simulink model "Stator_Resistance_tunning_induction_motor_NIKHIL_TYAGI"  (R2023b)
settings: Solver=ode4  StartTime=0.0  StopTime=5  RelTol=1e-3
libraries: spsabctoAlphaBetaZeroLib x3, spsStairGeneratorLib x3, slpidlib x3, spsThreePhaseVIMeasurementLib x2, spsAsynchronousMachineSIUnitsLib x1, spsSeriesRLCBranchLib x1, spsUniversalBridgeLib x1, spsThreePhaseSourceLib x1, spsSVPWMGenerator2LevelLib x1, spsTwoLevelConverterLib x1, spsVoltageMeasurementLib x1, spsdq0toabcLib x1
settings Model: Creator=tyagi  LastModifiedBy=tyagi_av27qbo
settings OptimizationCC: ReuseModelBlockBuffer=off

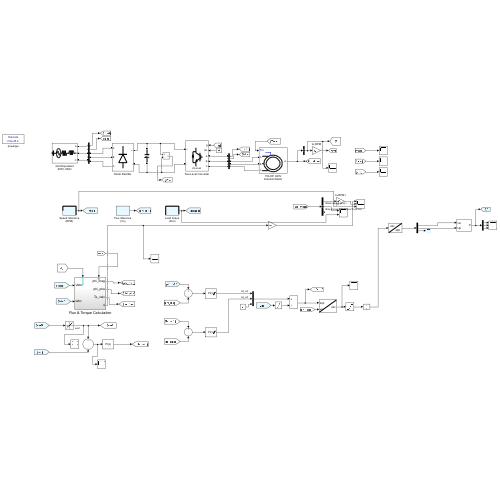
[thumbnail: Simulink's stored preview of the top-level diagram]
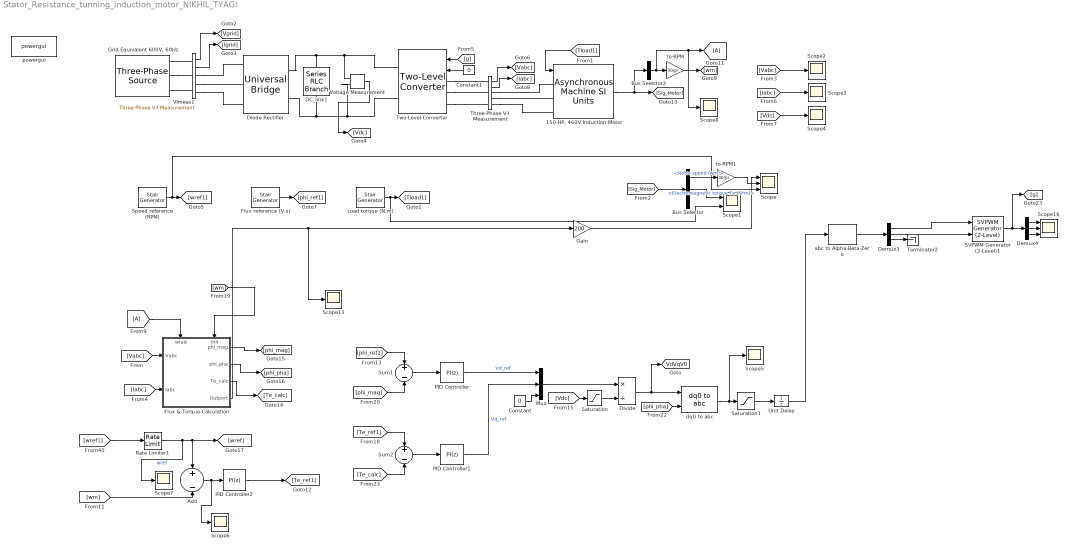
== system Stator_Resistance_tunning_induction_motor_NIKHIL_TYAGI ==
  "150-HP, 460V Induction Motor" : spsAsynchronousMachineSIUnitsLib/Asynchronous Machine SI Units  RotorType=Squirrel-cage  PresetModel=No  MechanicalLoad=Torque Tm  ShowDetailedParameters=on  ReferenceFrame=Stationary  Units=SI  MeasurementBus=off  NominalParameters="[ 111900  460  60]"  VoltageRatio=1  Stator=[0.0302,0.000283]  Rotor=[0.0302,0.000283]  Cage1=[ 0.022 0.226/377]  Cage2=[ 0.022 0.226/377]  Lm=0.01095  Mechanical=[2,0.02154,2]  PolePairs=2  InitialConditions=[1,0,0,0,0,0,0,0]  SimulateSaturation=off  Saturation=[0 0;0 0]  LoadFlowParameters=0  TsPowergui=0  TsBlock=-1  IterativeModel=Trapezoidal non iterative  IterativeDiscreteModel=Trapezoidal robust  Pmec=0  mask(Asynchronous Machine){}
      settings: AttributesFormatString=\n
  Add : Sum  Inputs=+|-
  Bus Selector : BusSelector  OutputSignals=Mechanical.Rotor speed (wm),Mechanical.Electromagnetic torque Te (N*m),Mechanical.Rotor angle thetam (rad)
  Bus Selector3 : BusSelector  OutputSignals=Mechanical.Rotor speed (wm)  OutputAsBus=on
  Constant : Constant  Value=0
  Constant1 : Constant  Value=0  SampleTime=2.5e-5
  DC_link1 : spsSeriesRLCBranchLib/Series RLC Branch  LConnTagsString=__new0  RConnTagsString=__new0  BranchType=C  Resistance=[]  Inductance=[]  SetiL0=off  InitialCurrent=0  Capacitance=0.02  Setx0=on  InitialVoltage=800  Measurements=None
  Demux3 : Demux  Outputs=3
  Demux4 : Demux  Outputs=3
  Diode Rectifier : spsUniversalBridgeLib/Universal Bridge  Arms=3  SnubberResistance=1e6  SnubberCapacitance=inf  Device=Diodes  Ron=1e-3  Lon=0  ForwardVoltages="[  0  0  ]"  ForwardVoltage=0  GTOparameters=[ 10e-6 , 20e-6 ]  IGBTparameters=[ 1e-6 , 2e-6 ]  Measurements=None  Measurements_2=None  converterType=Rectifier
  Divide : Product  Inputs=*/
  Flux & Torque Calculation : Subsystem
      settings: PortSchema="{\"entries\":[{\"content\":{\"sides\":[{\"content\":{\"connectorIds\":[\"In1\",\"In2\"]},\"type\":\"ConnectorPlacement.EquallySpacedRectSide\",\"uuid\":\"3523d87c-dc6a-4632-a5f5-d18ea8a44d5f\"},{\"content\":{\"connectorIds\":[\"Out1\",\"Out2\",\"Out3\",\"Out4\"],\"side\":\"RIGHT\"},\"type\":\"ConnectorPlacement.EquallySpacedRectSide\",\"uuid\":\"4f0e0cb3-79ce-4374-a058-bab3e7ce6c55\"},{\"content\":{\"connectorIds\":[\"In3\",\"In4\"],\"side\":\"TOP\"},\"type\":\"ConnectorPlacement.EquallySpacedRectSide\",\"uuid\":\"a4e44b10-f898-4bc5-ada3-d315e39bcfec\"}]},\"type\":\"ConnectorPlacement.EquallySpacedConnector\",\"uuid\":\"a05257d1-8fb8-45f9-88a8-3430eff1546f\"}],\"packageUris\":[\"http://schema.mathworks.com/mf0/Connector/R2020b\"],\"version\":\"1.0\"}"
  Flux reference (V.s) : spsStairGeneratorLib/Stair Generator  t=[0 3.5]  e=[0.89665,0.99628]  Ts=2.5e-5
  From9 : From
  Gain : Gain  Gain=200
  Goto11 : Goto
  "Grid Equivalent 600V, 60Hz" : spsThreePhaseSourceLib/Three-Phase Source  InternalConnection=Yg  VoltagePhases=off  Voltage=600  PhaseAngle=0  Voltage_phases=[25e3 25e3 25e3]/sqrt(3)  PhaseAngles_phases=[0 -120 +120]  Frequency=60  NonIdealSource=on  SpecifyImpedance=off  Resistance=0.01  Inductance=0.025e-3  ShortCircuitLevel=10e6  BaseVoltage=460  XRratio=5  BusType=swing  Pref=0  Qref=0  Prefabc=[10e3, 10e3, 10e3]  Qrefabc=[0, 0, 0]  Qmin=-inf  Qmax=inf
  Load torque (N.m) : spsStairGeneratorLib/Stair Generator  t=[0 1.5 2.0 ]  e=[0 500 50 ]  Ts=2.5e-5
  Mux : Mux  Inputs=3
  PID Controller : slpidlib/PID Controller  Controller=PI  Form=Parallel  TimeDomain=Discrete-time  UseExternalTs=off  SampleTime=2.5e-5  IntegratorMethod=Forward Euler  FilterMethod=Forward Euler  ControllerParametersSource=internal  P=650  I=8000  UseKiTs=off  D=0  N=100  UseFilter=on  TunerSelectOption=Transfer Function Based (PID Tuner App)  InitialConditionSource=internal  InitialConditionForIntegrator=0  InitialConditionForFilter=0  DifferentiatorICPrevScaledInput=0  ExternalReset=none  TrackingMode=off  Kt=1  LimitOutput=on  SatLimitsSource=internal  UpperSaturationLimit=900  LowerSaturationLimit=-900  LinearizeAsGain=on  AntiWindupMode=none  Kb=1  LimitIntegrator=off  UpperIntegratorSaturationLimit=inf  LowerIntegratorSaturationLimit=-inf  POutMin=[]  POutMax=[]  IOutMin=[]  IOutMax=[]  DOutMin=[]  DOutMax=[]  NOutMin=[]  NOutMax=[]  SumOutMin=[]  SumOutMax=[]  SaturationOutMin=[]  SaturationOutMax=[]  PParamMin=[]  PParamMax=[]  IParamMin=[]  IParamMax=[]  DParamMin=[]  DParamMax=[]  NParamMin=[]  NParamMax=[]  KbParamMin=[]  KbParamMax=[]  KtParamMin=[]  KtParamMax=[]  KbOutMin=[]  KbOutMax=[]  KtOutMin=[]  KtOutMax=[]  IntegratorOutMin=[]  IntegratorOutMax=[]  FilterOutMin=[]  FilterOutMax=[]  SumI1OutMin=[]  SumI1OutMax=[]  SumI2OutMin=[]  SumI2OutMax=[]  SumI3OutMin=[]  SumI3OutMax=[]  SumI4OutMin=[]  SumI4OutMax=[]  SumDOutMin=[]  SumDOutMax=[]  DifferentiatorOutMin=[]  DifferentiatorOutMax=[]  FilterDiffOutCoefMin=[]  FilterDiffOutCoefMax=[]  ReciprocalOutMin=[]  ReciprocalOutMax=[]  SumDenOutMin=[]  SumDenOutMax=[]  SumNumOutMin=[]  SumNumOutMax=[]  DivideOutMin=[]  DivideOutMax=[]  UdiffTsProdOutMin=[]  UdiffTsProdOutMax=[]  NTsProdOutMin=[]  NTsProdOutMax=[]  UintegralTsProdOutMin=[]  UintegralTsProdOutMax=[]  UngainTsProdOutMin=[]  UngainTsProdOutMax=[]  ClampingZeroOutDataTypeStr=Inherit: Inherit via back propagation  ClampingZeroOutMin=[]  ClampingZeroOutMax=[]  FilterDenConstantOutDataTypeStr=Inherit: Inherit via back propagation  FilterDenConstantOutMin=[]  FilterDenConstantOutMax=[]  PCopyOutDataTypeStr=Inherit: Inherit via back propagation  PCopyOutMin=[]  PCopyOutMax=[]  NCopyOutDataTypeStr=Inherit: Inherit via back propagation  NCopyOutMin=[]  NCopyOutMax=[]  IntegratorContinuousStateAttributes=''  IntegratorStateMustResolveToSignalObject=off  IntegratorRTWStateStorageClass=Auto  FilterContinuousStateAttributes=''  FilterStateMustResolveToSignalObject=off  FilterRTWStateStorageClass=Auto  ParallelPVariant=InternalParameters  IdealPVariant=Disabled  IVariant=InternalParameters  DVariant=Disabled  IntegratorVariant=Discrete  SatVariant=Enabled  AWVariant=Passthrough  PCopyVariant=Disabled  TRVariant=Disabled  FdbkBlocksVariant=Forward  IdealPFdbkVariant=Disabled  SatFdbkVariant=Disabled  DerivativeFilterVariant=Disabled  NVariant=Disabled  NCopyVariant=Disabled_SignalSpec  FilterICVariant=Disabled  IntegratorICVariant=InternalICs  ExternalResetVariant=Disabled  TRSumVariant=Passthrough  SumFdbkVariant=Disabled  SumVariant=Sum_PI  TsampFilterVariant=InternalTs  TsampNgainVariant=Passthrough  TsampIntegralVariant=Disabled_SignalSpec  ExternalSaturationOutDataTypeStr=Inherit: Same as second input
  PID Controller1 : slpidlib/PID Controller  Controller=PI  Form=Parallel  TimeDomain=Discrete-time  UseExternalTs=off  SampleTime=2.5e-5  IntegratorMethod=Forward Euler  FilterMethod=Forward Euler  ControllerParametersSource=internal  P=3  I=300  UseKiTs=off  D=0  N=100  UseFilter=on  TunerSelectOption=Transfer Function Based (PID Tuner App)  InitialConditionSource=internal  InitialConditionForIntegrator=0  InitialConditionForFilter=0  DifferentiatorICPrevScaledInput=0  ExternalReset=none  TrackingMode=off  Kt=1  LimitOutput=on  SatLimitsSource=internal  UpperSaturationLimit=900  LowerSaturationLimit=-900  LinearizeAsGain=on  AntiWindupMode=none  Kb=1  LimitIntegrator=off  UpperIntegratorSaturationLimit=inf  LowerIntegratorSaturationLimit=-inf  POutMin=[]  POutMax=[]  IOutMin=[]  IOutMax=[]  DOutMin=[]  DOutMax=[]  NOutMin=[]  NOutMax=[]  SumOutMin=[]  SumOutMax=[]  SaturationOutMin=[]  SaturationOutMax=[]  PParamMin=[]  PParamMax=[]  IParamMin=[]  IParamMax=[]  DParamMin=[]  DParamMax=[]  NParamMin=[]  NParamMax=[]  KbParamMin=[]  KbParamMax=[]  KtParamMin=[]  KtParamMax=[]  KbOutMin=[]  KbOutMax=[]  KtOutMin=[]  KtOutMax=[]  IntegratorOutMin=[]  IntegratorOutMax=[]  FilterOutMin=[]  FilterOutMax=[]  SumI1OutMin=[]  SumI1OutMax=[]  SumI2OutMin=[]  SumI2OutMax=[]  SumI3OutMin=[]  SumI3OutMax=[]  SumI4OutMin=[]  SumI4OutMax=[]  SumDOutMin=[]  SumDOutMax=[]  DifferentiatorOutMin=[]  DifferentiatorOutMax=[]  FilterDiffOutCoefMin=[]  FilterDiffOutCoefMax=[]  ReciprocalOutMin=[]  ReciprocalOutMax=[]  SumDenOutMin=[]  SumDenOutMax=[]  SumNumOutMin=[]  SumNumOutMax=[]  DivideOutMin=[]  DivideOutMax=[]  UdiffTsProdOutMin=[]  UdiffTsProdOutMax=[]  NTsProdOutMin=[]  NTsProdOutMax=[]  UintegralTsProdOutMin=[]  UintegralTsProdOutMax=[]  UngainTsProdOutMin=[]  UngainTsProdOutMax=[]  ClampingZeroOutDataTypeStr=Inherit: Inherit via back propagation  ClampingZeroOutMin=[]  ClampingZeroOutMax=[]  FilterDenConstantOutDataTypeStr=Inherit: Inherit via back propagation  FilterDenConstantOutMin=[]  FilterDenConstantOutMax=[]  PCopyOutDataTypeStr=Inherit: Inherit via back propagation  PCopyOutMin=[]  PCopyOutMax=[]  NCopyOutDataTypeStr=Inherit: Inherit via back propagation  NCopyOutMin=[]  NCopyOutMax=[]  IntegratorContinuousStateAttributes=''  IntegratorStateMustResolveToSignalObject=off  IntegratorRTWStateStorageClass=Auto  FilterContinuousStateAttributes=''  FilterStateMustResolveToSignalObject=off  FilterRTWStateStorageClass=Auto  ParallelPVariant=InternalParameters  IdealPVariant=Disabled  IVariant=InternalParameters  DVariant=Disabled  IntegratorVariant=Discrete  SatVariant=Enabled  AWVariant=Passthrough  PCopyVariant=Disabled  TRVariant=Disabled  FdbkBlocksVariant=Forward  IdealPFdbkVariant=Disabled  SatFdbkVariant=Disabled  DerivativeFilterVariant=Disabled  NVariant=Disabled  NCopyVariant=Disabled_SignalSpec  FilterICVariant=Disabled  IntegratorICVariant=InternalICs  ExternalResetVariant=Disabled  TRSumVariant=Passthrough  SumFdbkVariant=Disabled  SumVariant=Sum_PI  TsampFilterVariant=InternalTs  TsampNgainVariant=Passthrough  TsampIntegralVariant=Disabled_SignalSpec  ExternalSaturationOutDataTypeStr=Inherit: Same as second input
  PID Controller2 : slpidlib/PID Controller  Controller=PI  Form=Parallel  TimeDomain=Discrete-time  UseExternalTs=off  SampleTime=2.5e-5  IntegratorMethod=Forward Euler  FilterMethod=Forward Euler  ControllerParametersSource=internal  P=60  I=600  UseKiTs=off  D=0  N=100  UseFilter=on  TunerSelectOption=Transfer Function Based (PID Tuner App)  InitialConditionSource=internal  InitialConditionForIntegrator=0  InitialConditionForFilter=0  DifferentiatorICPrevScaledInput=0  ExternalReset=none  TrackingMode=off  Kt=1  LimitOutput=off  SatLimitsSource=internal  UpperSaturationLimit=inf  LowerSaturationLimit=-inf  LinearizeAsGain=on  AntiWindupMode=none  Kb=1  LimitIntegrator=off  UpperIntegratorSaturationLimit=inf  LowerIntegratorSaturationLimit=-inf  POutMin=[]  POutMax=[]  IOutMin=[]  IOutMax=[]  DOutMin=[]  DOutMax=[]  NOutMin=[]  NOutMax=[]  SumOutMin=[]  SumOutMax=[]  SaturationOutMin=[]  SaturationOutMax=[]  PParamMin=[]  PParamMax=[]  IParamMin=[]  IParamMax=[]  DParamMin=[]  DParamMax=[]  NParamMin=[]  NParamMax=[]  KbParamMin=[]  KbParamMax=[]  KtParamMin=[]  KtParamMax=[]  KbOutMin=[]  KbOutMax=[]  KtOutMin=[]  KtOutMax=[]  IntegratorOutMin=[]  IntegratorOutMax=[]  FilterOutMin=[]  FilterOutMax=[]  SumI1OutMin=[]  SumI1OutMax=[]  SumI2OutMin=[]  SumI2OutMax=[]  SumI3OutMin=[]  SumI3OutMax=[]  SumI4OutMin=[]  SumI4OutMax=[]  SumDOutMin=[]  SumDOutMax=[]  DifferentiatorOutMin=[]  DifferentiatorOutMax=[]  FilterDiffOutCoefMin=[]  FilterDiffOutCoefMax=[]  ReciprocalOutMin=[]  ReciprocalOutMax=[]  SumDenOutMin=[]  SumDenOutMax=[]  SumNumOutMin=[]  SumNumOutMax=[]  DivideOutMin=[]  DivideOutMax=[]  UdiffTsProdOutMin=[]  UdiffTsProdOutMax=[]  NTsProdOutMin=[]  NTsProdOutMax=[]  UintegralTsProdOutMin=[]  UintegralTsProdOutMax=[]  UngainTsProdOutMin=[]  UngainTsProdOutMax=[]  ClampingZeroOutDataTypeStr=Inherit: Inherit via back propagation  ClampingZeroOutMin=[]  ClampingZeroOutMax=[]  FilterDenConstantOutDataTypeStr=Inherit: Inherit via back propagation  FilterDenConstantOutMin=[]  FilterDenConstantOutMax=[]  PCopyOutDataTypeStr=Inherit: Inherit via back propagation  PCopyOutMin=[]  PCopyOutMax=[]  NCopyOutDataTypeStr=Inherit: Inherit via back propagation  NCopyOutMin=[]  NCopyOutMax=[]  IntegratorContinuousStateAttributes=''  IntegratorStateMustResolveToSignalObject=off  IntegratorRTWStateStorageClass=Auto  FilterContinuousStateAttributes=''  FilterStateMustResolveToSignalObject=off  FilterRTWStateStorageClass=Auto  ParallelPVariant=InternalParameters  IdealPVariant=Disabled  IVariant=InternalParameters  DVariant=Disabled  IntegratorVariant=Discrete  SatVariant=Disabled  AWVariant=Passthrough  PCopyVariant=Disabled  TRVariant=Disabled  FdbkBlocksVariant=Forward  IdealPFdbkVariant=Disabled  SatFdbkVariant=Disabled  DerivativeFilterVariant=Disabled  NVariant=Disabled  NCopyVariant=Disabled_SignalSpec  FilterICVariant=Disabled  IntegratorICVariant=InternalICs  ExternalResetVariant=Disabled  TRSumVariant=Passthrough  SumFdbkVariant=Disabled  SumVariant=Sum_PI  TsampFilterVariant=InternalTs  TsampNgainVariant=Passthrough  TsampIntegralVariant=Disabled_SignalSpec  ExternalSaturationOutDataTypeStr=Inherit: Same as second input
  Rate Limiter1 : RateLimiter  RisingSlewLimit=1200  FallingSlewLimit=-1200  SampleTimeMode=inherited  LinearizeAsGain=off
  SVPWM Generator (2-Level)1 : spsSVPWMGenerator2LevelLib/SVPWM Generator (2-Level)  InputType=alpha-beta components  SwitchingPattern=Pattern #1  Fc=2000  ParUref=[0.8 -30 50]  Ts=0
  Saturation : Saturate  UpperLimit=inf  LowerLimit=eps
  Saturation1 : Saturate  UpperLimit=2/sqrt(3)  LowerLimit=-2*sqrt(3)
  Scope : Scope  NumInputPorts=3
  Scope1 : Scope  NumInputPorts=2
  Scope{2..8,13} (8 alike) : Scope
  Scope16 : Scope  NumInputPorts=3
  Speed reference (RPM) : spsStairGeneratorLib/Stair Generator  t=[0 0.1 2.5]  e=[0 500 -500]  Ts=2.5e-5
  Sum1 : Sum  Inputs=+-  InputSameDT=on  SaturateOnIntegerOverflow=on  OutDataTypeStr=Inherit: Same as first input
  Sum2 : Sum  Inputs=+-  InputSameDT=on  SaturateOnIntegerOverflow=on  OutDataTypeStr=Inherit: Same as first input
  Terminator2 : Terminator
  Three-Phase V-I Measurement : spsThreePhaseVIMeasurementLib/Three-Phase V-I Measurement  VoltageMeasurement=phase-to-phase  SetLabelV=off  LabelV=Vabc  Vpu=off  VpuLL=off  CurrentMeasurement=yes  SetLabelI=off  LabelI=Iabc  Ipu=off  Pbase=100e6  Vbase=500e3  OutputType=Complex  PhasorSimulation=off  PSBequivalent=0
  Two-Level Converter : spsTwoLevelConverterLib/Two-Level Converter  ModelType=Switching function  Ron=1e-3  Rs=1e6  Cs=inf  Vforward=[0,0]  Ron_Diode=1e-3  Rs_Diode=1e6  Cs_Diode=inf  Vf_Diode=0  Rs_CurrentSource=inf  Ron_ACsource=1e-3
  Unit Delay : UnitDelay  SampleTime=-1  HasFrameUpgradeWarning=on
  VImeas1 : spsThreePhaseVIMeasurementLib/Three-Phase V-I Measurement  VoltageMeasurement=phase-to-ground  SetLabelV=off  LabelV=Vabc  Vpu=off  VpuLL=off  CurrentMeasurement=yes  SetLabelI=off  LabelI=Iabc  Ipu=off  Pbase=100e6  Vbase=500e3  OutputType=Complex  PhasorSimulation=off  PSBequivalent=0
  Voltage Measurement : spsVoltageMeasurementLib/Voltage Measurement  PhasorSimulation=off  OutputType=Complex  PSBequivalent=0
  abc to Alpha-Beta-Zero : spsabctoAlphaBetaZeroLib/abc to Alpha-Beta-Zero
  dq0 to abc : spsdq0toabcLib/dq0 to abc  Alignment=Aligned with phase A axis
  powergui : spspowerguiLib/powergui  Priority=2  SimulationMode=Discrete  SampleTime=2.5e-5  frequency=60  Iterations=50  frequencyindice=0  Pbase=100e6  ErrMax=1e-4  UnitsV=kV  UnitsW=MW  buscounter=0  FunctionMessages=off  echomessages=off  EnableUseOfTLC=off  CurrentSourceSwitches=off  DisableSnubberDevices=off  DisableRonSwitches=off  DisableVfSwitches=off  DisplayEquations=off  AutomaticDiscreteSolvers=off  SolverType=Tustin/Backward Euler (TBE)  Interpol=off  ExternalGateDelay=off  methode=off  Ts=0  x0status=blocks  SPID=off  SwTol=0  HookPort=off  NonlinearTolerance=1e-4  nMaxIteration=100  ContinueOnMaxIteration=on  RestoreLinks=warning  ResistiveCurrentMeasurement=off  Frange=[0:2:500]  Ylog=off  Xlog=on  ShowGrid=off  save=off  variable=ZData  structure=ScopeData_Vabc_Motor  ZoomFFT=off  StartTime=3.9  cycles=1  DisplayStyle=1  fundamental=22  FreqAxis=off  MaxFrequency=1000  frequencyindicesteady=1  RmsSteady=1  display=off
  to-RPM : Gain  Gain=30/pi
  to-RPM1 : Gain  Gain=30/pi
  tag scope: VdVqV0=global
  wires:
  [Tload1] -> "150-HP, 460V Induction Motor"/1
  Voltage Measurement/1 -> [Vdc]
  "150-HP, 460V Induction Motor"/1 -> [Sig_Motor], Bus Selector3/1
  VImeas1/1 -> [Vgrid]
  Three-Phase V-I Measurement/1 -> [Vabc]
  Constant1/1 -> Two-Level Converter/2
  Flux reference (V.s)/1 -> [phi_ref1]
  [g] -> Two-Level Converter/1
  Load torque (N.m)/1 -> Scope1/2, [Tload1]
  Three-Phase V-I Measurement/2 -> [Iabc]
  Speed reference (RPM)/1 -> Scope/3, [wref1]
  VImeas1/2 -> [Igrid]
  to-RPM/1 -> [wm]
  Unit Delay/1 -> abc to Alpha-Beta-Zero/1
  Bus Selector3/1 -> Goto11/1, Scope8/1, to-RPM/1
  [wm] -> Add/2
  PID Controller1/1 -> Mux/2  "Vq_ref"
  Sum2/1 -> PID Controller1/1
  Add/1 -> Scope6/1, PID Controller2/1
  Sum1/1 -> PID Controller/1
  [Vdc] -> Saturation/1
  Mux/1 -> Divide/1
  [Iabc] -> Flux & Torque Calculation/2(Iabc)
  PID Controller2/1 -> [Te_ref1]
  [Vabc] -> Flux & Torque Calculation/1(Vabc)
  [Te_ref1] -> Sum2/1
  Saturation1/1 -> Unit Delay/1
  Flux & Torque Calculation/1(phi_mag) -> [phi_mag]
  Divide/1 -> dq0 to abc/1, [VdVqV0]
  [phi_ref1] -> Sum1/1
  [wref1] -> Rate Limiter1/1
  Rate Limiter1/1 -> Scope7/1, [wref], Add/1  "wref"
  Constant/1 -> Mux/3
  dq0 to abc/1 -> Scope5/1, Saturation1/1
  [phi_pha] -> dq0 to abc/2
  Flux & Torque Calculation/2(phi_pha) -> [phi_pha]
  [phi_mag] -> Sum1/2
  [Te_calc] -> Sum2/2
  Flux & Torque Calculation/3(Te_calc) -> [Te_calc]
  PID Controller/1 -> Mux/1  "Vd_ref"
  Saturation/1 -> Divide/2
  [Sig_Motor] -> Bus Selector/1
  Bus Selector/1 -> to-RPM1/1  "<Rotor speed (wm)>"
  Bus Selector/2 -> Scope1/1  "<Electromagnetic torque Te (N*m)>"
  [Vabc] -> Scope2/1
  [Iabc] -> Scope3/1
  [Vdc] -> Scope4/1
  to-RPM1/1 -> Scope/2
  From9/1 -> Flux & Torque Calculation/3(wrad)
  abc to Alpha-Beta-Zero/1 -> Demux3/1
  Demux3/1 -> SVPWM Generator (2-Level)1/1
  Demux3/2 -> SVPWM Generator (2-Level)1/2
  SVPWM Generator (2-Level)1/1 -> [g], Demux4/1
  Demux4/1 -> Scope16/1
  Demux4/2 -> Scope16/2
  Demux4/3 -> Scope16/3
  Demux3/3 -> Terminator2/1
  [wm] -> Flux & Torque Calculation/4(In4)
  Flux & Torque Calculation/4(Outport) -> Scope13/1, Gain/1
  Gain/1 -> Scope/1
  connections:
  Two-Level Converter/RConn2 -- Voltage Measurement/LConn2 -- Diode Rectifier/RConn2 -- DC_link1/RConn1
  "Grid Equivalent 600V, 60Hz"/RConn2 -- VImeas1/LConn2
  Two-Level Converter/LConn2 -- Three-Phase V-I Measurement/LConn2
  Two-Level Converter/LConn3 -- Three-Phase V-I Measurement/LConn3
  "Grid Equivalent 600V, 60Hz"/RConn1 -- VImeas1/LConn1
  Three-Phase V-I Measurement/RConn3 -- "150-HP, 460V Induction Motor"/LConn3
  "Grid Equivalent 600V, 60Hz"/RConn3 -- VImeas1/LConn3
  VImeas1/RConn3 -- Diode Rectifier/LConn3
  VImeas1/RConn2 -- Diode Rectifier/LConn2
  VImeas1/RConn1 -- Diode Rectifier/LConn1
  Two-Level Converter/LConn1 -- Three-Phase V-I Measurement/LConn1
  Three-Phase V-I Measurement/RConn1 -- "150-HP, 460V Induction Motor"/LConn1
  Three-Phase V-I Measurement/RConn2 -- "150-HP, 460V Induction Motor"/LConn2
  DC_link1/LConn1 -- Diode Rectifier/RConn1 -- Voltage Measurement/LConn1 -- Two-Level Converter/RConn1

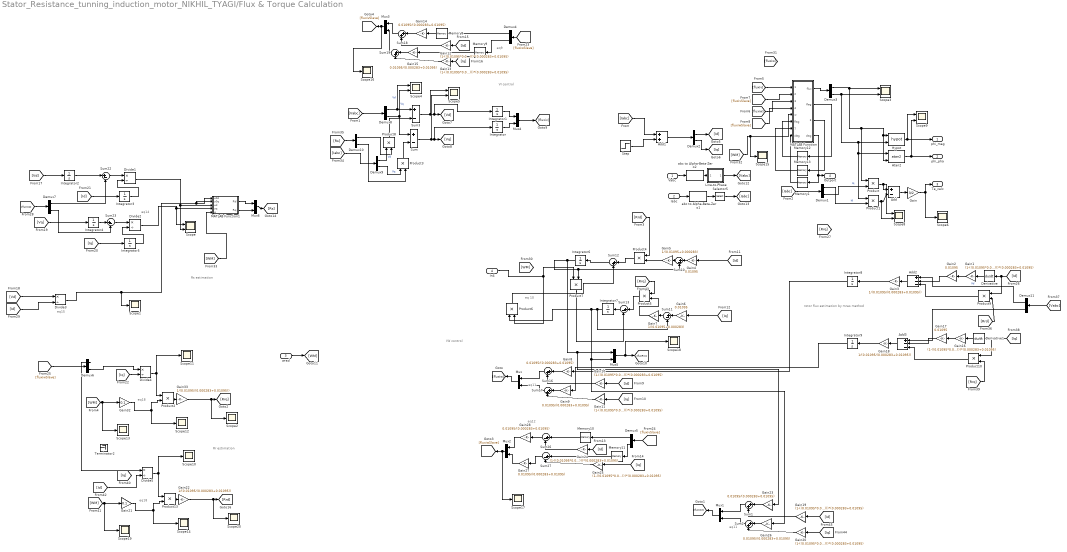
== system Stator_Resistance_tunning_induction_motor_NIKHIL_TYAGI/Flux & Torque Calculation ==
  note: rotor flux estimation by mras method
  note: Rr estimation
  note: Rs estimation
  note: VI control
  note: IW control
  note: eq
      | 10
  note: eq11
  note: eq9
  note: eq12
  note: eq15
  note: eq18
  note: eq14
  note: eq18
  note: eq11
  Vabc : Inport  PortDimensions=3
  Iabc : Inport  Port=2  PortDimensions=3
  wrad : Inport  Port=3
  In4 : Inport  Port=4
  Add : Sum  Inputs=+-
  Add1 : Sum
  Add2 : Sum  Inputs=+--
  Add3 : Sum  Inputs=+--
  Atan2 : Trigonometry  Operator=atan2
  Demux{1..11} (11 alike) : Demux  Outputs=2
  Derivative : Derivative
  Derivative1 : Derivative
  Divide{1..5} (5 alike) : Product  Inputs=*/
  Gain : Gain  Gain=3/2
  Gain{1,10..13,16,19..20,24..25} (10 alike) : Gain  Gain=(1-((0.01095*0.01095)/((0.000283+0.01095)*(0.01095+0.000283))))*(0.000283+0.01095)
  Gain{8..9,14..15,23,26..28} (8 alike) : Gain  Gain=0.01095/(0.000283+0.01095)
  Gain{2,4,6,17} (4 alike) : Gain  Gain=0.01095
  Gain{3,18,22,33} (4 alike) : Gain  Gain=1/(0.01095/(0.000283+0.01095))
  Gain21 : Gain  Gain=0.1
  Gain32 : Gain  Gain=0.1
  Gain5 : Gain  Gain=1/(0.01095+0.000283)
  Gain7 : Gain  Gain=1/(0.01095+0.000283)
  Hypot : Math  Operator=hypot
  Integrator{,1..9} (10 alike) : Integrator
  Line-to-Phase : Subsystem
  MATLAB Function : MATLAB Function  TreatAsAtomicUnit=on
  MATLAB Function1 : MATLAB Function  TreatAsAtomicUnit=on
  Memory{1,8..13} (7 alike) : Memory
  Mux{,1..6} (7 alike) : Mux  Inputs=2
  Product{,1..10,13} (12 alike) : Product
  Scope{,3..5,8..9} (6 alike) : Scope  NumInputPorts=2
  Scope{1..2,6,10..20} (14 alike) : Scope
  Selector5 : Selector  InputPortWidth=3  IndexOptions=Index vector (dialog)  Indices=[1,2]  OutputSizes=1
  Step : Step  Time=0.001  Before=[1,1]  After=0  SampleTime=0
  Sum : Sum  Inputs=+-  InputSameDT=on  SaturateOnIntegerOverflow=on  OutDataTypeStr=Inherit: Same as first input
  Sum{1..2,12,16..19} (7 alike) : Sum  Inputs=|++
  Sum{10..11,13,22..23,26..27} (7 alike) : Sum  Inputs=|+-
  Sum3 : Sum  Inputs=+-  InputSameDT=on  SaturateOnIntegerOverflow=on  OutDataTypeStr=Inherit: Same as first input
  Terminator2 : Terminator
  abc to Alpha-Beta-Zero1 : spsabctoAlphaBetaZeroLib/abc to Alpha-Beta-Zero
  abc to Alpha-Beta-Zero2 : spsabctoAlphaBetaZeroLib/abc to Alpha-Beta-Zero
  phi_mag : Outport
  phi_pha : Outport  Port=2
  Te_calc : Outport  Port=3
  Outport : Outport  Port=4
  wires:
  Line-to-Phase/1(PhaseV) -> [Vabc]
  abc to Alpha-Beta-Zero2/1 -> Line-to-Phase/1(LineV)
  Vabc/1 -> abc to Alpha-Beta-Zero2/1
  Demux1/2 -> Product/2  "Iq"
  Demux1/1 -> Product1/2  "Id"
  Gain/1 -> Te_calc/1, Scope6/1
  Hypot/1 -> Scope9/1, phi_mag/1
  Atan2/1 -> Scope9/2, phi_pha/1
  Product3/1 -> Sum/2
  abc to Alpha-Beta-Zero1/1 -> Selector5/1
  Iabc/1 -> abc to Alpha-Beta-Zero1/1
  Product/1 -> Scope8/1, Add/1
  Product1/1 -> Scope8/2, Add/2
  Add/1 -> Gain/1
  [Id] -> Gain4/1
  Gain6/1 -> Sum11/1
  Sum10/1 -> Gain5/1
  Sum11/1 -> Gain7/1
  Product6/1 -> Sum12/2
  Gain5/1 -> Product4/2
  [Iq] -> Gain6/1
  Gain7/1 -> Product5/2
  Sum13/1 -> Integrator7/1
  Gain4/1 -> Sum10/1
  Gain10/1 -> Sum16/2
  Gain11/1 -> Sum17/2
  Gain9/1 -> Sum17/1
  Gain8/1 -> Sum16/1
  Gain13/1 -> Sum19/2
  Gain15/1 -> Sum19/1
  Gain14/1 -> Sum18/1
  Gain12/1 -> Sum18/2
  Memory9/1 -> Gain15/1
  Memory8/1 -> Gain14/1
  Sum19/1 -> Mux3/2
  Gain24/1 -> Sum26/2
  Gain25/1 -> Sum27/2
  Sum26/1 -> Gain28/1
  Sum27/1 -> Gain27/1
  Memory10/1 -> Sum26/1
  Sum18/1 -> Mux3/1
  Memory11/1 -> Sum27/1
  Integrator3/1 -> Divide1/2
  Product2/1 -> Gain33/1
  Gain28/1 -> Mux2/1
  Divide4/1 -> Product2/1, Scope11/1
  Demux2/2 -> [Iq]
  Integrator5/1 -> Divide2/2
  Sum23/1 -> Divide2/1
  Sum22/1 -> Divide1/1
  Integrator2/1 -> Sum22/1
  Demux2/1 -> [Id]
  Gain32/1 -> Product2/2, Scope12/1
  Sum16/1 -> Mux/1
  Integrator4/1 -> Sum23/1
  Sum17/1 -> Mux/2
  Gain27/1 -> Mux2/2
  Mux/1 -> [fluxiw]
  Demux3/1 -> Atan2/2, Hypot/1, Product/1, Scope3/1
  Demux3/2 -> Hypot/2, Atan2/1, Product1/1, Scope3/2
  Divide3/1 -> MATLAB Function1/1(u0d), MATLAB Function1/2(u0q), Scope1/1
  wrad/1 -> [WM]
  Product4/1 -> Sum12/1
  Product5/1 -> Sum13/1
  Mux2/1 -> Scope17/1, [fluxiwSlave]
  Mux3/1 -> Scope16/1, [fluxivSlave]
  [fluxivSlave] -> MATLAB Function/2(fluxIVslave)
  [fluxiw] -> MATLAB Function/3(fluxIW)
  [fluxiwSlave] -> MATLAB Function/4(FluxIWslave)
  [Id] -> Gain10/1
  [Iq] -> Gain11/1
  [Id] -> Gain24/1
  [Iq] -> Gain25/1
  [Id] -> Gain12/1
  [Iq] -> Gain13/1
  [Vd] -> Integrator2/1
  [Vd] -> Divide3/1
  [Iq] -> Integrator5/1
  [Id] -> Integrator3/1
  [Iq] -> Divide4/2
  [fluxiwSlave] -> Demux4/1
  Demux4/1 -> Memory8/1
  Demux4/2 -> Memory9/1
  [fluxivSlave] -> Demux5/1
  Demux5/1 -> Memory10/1
  Demux5/2 -> Memory11/1
  [fluxiwSlave] -> Demux6/1
  Demux6/2 -> Divide4/1
  [fluxiw2] -> Demux7/1
  Demux7/1 -> Sum22/2
  Demux7/2 -> Sum23/2
  [Id] -> Divide3/2
  MATLAB Function/2(flag) -> Memory12/1
  MATLAB Function/3(mlag) -> Memory13/1
  Memory12/1 -> MATLAB Function/6("flag ")
  Memory13/1 -> MATLAB Function/7("mlag ")
  Selector5/1 -> [Iabc]
  Step/1 -> Add1/2
  Demux8/1 -> Scope4/1, Sum3/1  "Vd"
  Demux8/2 -> Sum/1, Scope4/2  "Vq"
  Sum3/1 -> Scope5/1, Integrator1/1, [Vd]
  Sum/1 -> Scope5/2, Integrator/1, [Vq]
  Product8/1 -> Sum3/2
  Demux9/1 -> Product8/1  "Vd"
  Demux9/2 -> Product3/1  "Vq"
  Divide1/1 -> Scope/2, MATLAB Function1/3(ud)
  Divide2/1 -> Scope/1, MATLAB Function1/4(uq)
  Integrator1/1 -> Mux4/1
  Integrator/1 -> Mux4/2
  Mux4/1 -> [fluxiv]
  Sum12/1 -> Integrator6/1
  Integrator6/1 -> Gain23/1, Mux5/1, Product7/2, Sum10/2
  Integrator7/1 -> Sum11/2, Gain26/1, Mux5/2, Product6/1
  Product7/1 -> Sum13/2
  [Vq] -> Integrator4/1
  Add1/1 -> Demux2/1
  MATLAB Function1/1(Rd) -> Mux6/1
  MATLAB Function1/2(Rq) -> Mux6/2
  Gain33/1 -> Scope2/1, [Rrq]
  Mux5/1 -> Scope18/1, [fluxRiw]
  [WM] -> Scope13/1, Gain32/1
  In4/1 -> Product7/1, Product6/2
  [WM] -> MATLAB Function/5(w), Scope15/1
  [WM] -> MATLAB Function1/5(w)
  [Vabc] -> Demux8/1
  [Iabc] -> Demux9/1
  Mux6/1 -> [Rs]
  [Rs] -> Demux10/1
  Demux10/1 -> Product8/2
  Demux10/2 -> Product3/2
  [Iabc] -> Add1/1
  [Iabc] -> Demux1/1
  [fluxiv] -> MATLAB Function/1(fluxIV)
  [WM] -> Scope19/1, Gain21/1
  Divide5/1 -> Product13/1, Scope10/1
  Gain22/1 -> Scope20/1, [Rrd]
  Demux6/1 -> Divide5/1
  Product13/1 -> Gain22/1
  [Id] -> Divide5/2
  Gain21/1 -> Product13/2, Scope14/1
  [Rrd] -> Product4/1
  [Rrq] -> Product5/1
  [Id] -> Product9/1, Derivative/1
  Derivative/1 -> Gain1/1
  Gain1/1 -> Gain2/1
  [Rrd] -> Product9/2
  [Vabc] -> Demux11/1
  Demux11/1 -> Add2/1  "Vd"
  Gain2/1 -> Add2/2
  Product9/1 -> Add2/3
  Add2/1 -> Gain3/1
  Gain3/1 -> Integrator8/1
  [Iq] -> Product10/1, Derivative1/1
  Demux11/2 -> Add3/1
  Gain17/1 -> Add3/2
  [Rrq] -> Product10/2
  Add3/1 -> Gain18/1
  Product10/1 -> Add3/3
  Derivative1/1 -> Gain16/1
  Gain16/1 -> Gain17/1
  Gain18/1 -> Integrator9/1
  Integrator8/1 -> Gain8/1
  Integrator9/1 -> Gain9/1
  MATLAB Function/4(clag) -> Outport/1, Memory1/1
  Memory1/1 -> MATLAB Function/8("clag ")
  Mux1/1 -> [fluxiw2]
  Sum2/1 -> Mux1/2
  [Id] -> Gain19/1
  Sum1/1 -> Mux1/1
  Gain23/1 -> Sum1/1
  Gain26/1 -> Sum2/1
  Gain20/1 -> Sum2/2
  Gain19/1 -> Sum1/2
  [Iq] -> Gain20/1
  MATLAB Function/1(flux) -> Demux3/1

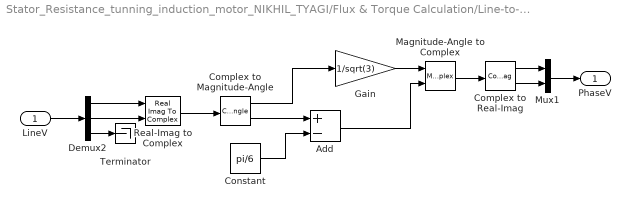
== system Stator_Resistance_tunning_induction_motor_NIKHIL_TYAGI/Flux & Torque Calculation/Line-to-Phase ==
  LineV : Inport
  Add : Sum  Inputs=+-
  Complex to Magnitude-Angle : ComplexToMagnitudeAngle
  Complex to Real-Imag : ComplexToRealImag
  Constant : Constant  Value=pi/6
  Demux2 : Demux  Outputs=3
  Gain : Gain  Gain=1/sqrt(3)
  Magnitude-Angle to Complex : MagnitudeAngleToComplex
  Mux1 : Mux  Inputs=2
  Real-Imag to Complex : RealImagToComplex
  Terminator : Terminator
  PhaseV : Outport
  wires:
  LineV/1 -> Demux2/1
  Demux2/3 -> Terminator/1
  Demux2/2 -> Real-Imag to Complex/2
  Real-Imag to Complex/1 -> Complex to Magnitude-Angle/1
  Demux2/1 -> Real-Imag to Complex/1
  Complex to Real-Imag/2 -> Mux1/2
  Magnitude-Angle to Complex/1 -> Complex to Real-Imag/1
  Constant/1 -> Add/2
  Complex to Real-Imag/1 -> Mux1/1
  Complex to Magnitude-Angle/2 -> Add/1
  Mux1/1 -> PhaseV/1
  Add/1 -> Magnitude-Angle to Complex/2
  Gain/1 -> Magnitude-Angle to Complex/1
  Complex to Magnitude-Angle/1 -> Gain/1

== matlab function Stator_Resistance_tunning_induction_motor_NIKHIL_TYAGI/Flux & Torque Calculation/MATLAB Function ==
  data: fluxIV input; flux output; fluxIVslave input; fluxIW input; FluxIWslave input; w input; flag input; mlag input; flag output; mlag output; clag input; clag output
function [flux,flag,mlag,clag]= fcn(fluxIV,fluxIVslave,fluxIW,FluxIWslave,w,flag,mlag,clag)
if isempty(flag)
    flag=1;
    mlag=1;
    clag=1
end
if w>=20 || w<=-20
    clag=0;
%     if flag==1
%         flux=fluxIVslave;
%         flag=0;
%     else
        flux=fluxIV;
        flag=0;
        mlag=1;
%     end
elseif w<20 || w>-20
    clag=1
%     if mlag==1
%         flux=FluxIWslave;
%         mlag=0;
%     else
        flux=fluxIW;
        mlag=0;
        flag=1;
%     end
else
    flux=[0 
          0];
end

== matlab function Stator_Resistance_tunning_induction_motor_NIKHIL_TYAGI/Flux & Torque Calculation/MATLAB Function1 ==
  data: u0d input; Rd output; u0q input; ud input; uq input; w input; Rq output
function [Rd,Rq]= fcn(u0d,u0q,ud,uq,w)

if w==0
    Rd=u0d;
    Rq=u0q;
elseif w>0.01 || w<-0.01
    Rd=ud;
    Rq=uq;
else
    Rd=0.0302;
    Rq=0.0302;
end
